simulink model "test_nlin_interp2"  (R2015a)
settings: Solver=ode45  StartTime=0.0  StopTime=u(end,1)  FixedStep=0.001  RelTol=1e-6
PostLoadFcn:
  | , if any(exist('dsrtsu_mdlpostloadfcn', 'file') == [2, 3, 6]), try dsrtsu_mdlpostloadfcn('Execute', bdroot); catch fprintf('Error in PostLoadFcn (dsrtsu_mdlpostloadfcn) for model "%s":\n %s\n', bdroot, lasterr); end, end,
values from neighbouring files (symbols this model uses):
  c = rectangle('Parent',ax)    [DoublePendulum.m]    (also in init.m = 2.99880047981; interpolate.m = 2.99880047981; plot_17.m = 2.99880047981)
  g = 9.81    [init.m]    (also in interpolate.m; plot_17.m; plot_generic.m)
  T1 = 0.0395    [init.m]    (also in interpolate.m = 0.025; plot_17.m = 0.025; plot_generic.m)
settings Model: DSRTSU_INTERNAL_RTI_VER=360  DSRTSU_INTERNAL_RTI_TYPE=rti1104  CovSFcnEnable=off  Creator=labor  LastModifiedBy=Schuettler
settings DataIOCC: LimitDataPoints=off  SignalLoggingSaveFormat=ModelDataLogs
settings OptimizationCC: BlockReduction=off  OptimizeBlockIOStorage=off  BufferReuse=off  GlobalBufferReuse=off  ExpressionFolding=off  ExpressionDepthLimit=2147483647  LocalBlockOutputs=off  InitFltsAndDblsToZero=on  OptimizeModelRefInitCode=on  LifeSpan=1
settings DebuggingCC: UnderspecifiedInitializationDetection=Classic  MergeDetectMultiDrivingBlocksExec=none  SolverPrmCheckMsg=warning  FcnCallInpInsideContextMsg=UseLocalSettings  StateNameClashWarn=warning
settings HardwareCC: ProdIntDivRoundTo=Zero  ProdEndianess=BigEndian  ProdHWDeviceType=Generic->Custom  TargetIntDivRoundTo=Zero  TargetEndianess=BigEndian  TargetHWDeviceType=Generic->Custom
settings RTWCC: SystemTargetFile=ert.tlc  TemplateMakefile=ert_default_tmf  Description=Embedded Coder
settings CodeAppCC: IgnoreCustomStorageClasses=off
settings ERTTargetCC: ParMdlRefBuildCompliant=on  CompOptLevelCompliant=on  ConcurrentExecutionCompliant=on  ERTFirstTimeCompliant=on  SupportContinuousTime=off  SupportVariableSizeSignals=off  ModelStepFunctionPrototypeControlCompliant=on  CPPClassGenCompliant=on  InlinedParameterPlacement=Hierarchical  ERTCustomFileTemplate=example_file_process.tlc

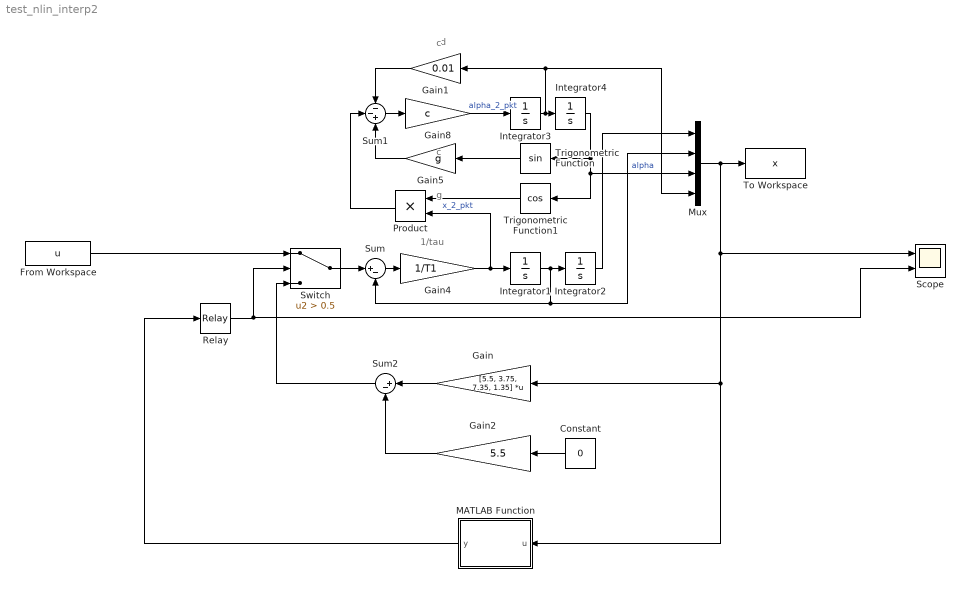
== system test_nlin_interp2 ==
  note: d
  note: 1/tau
  note: g
  note: c
  note: c
  Constant : Constant  Value=0
  From Workspace : FromWorkspace  VariableName=u  SampleTime=0
  Gain : Gain  Gain=[5.5, 3.75, 7.35, 1.35]  Multiplication=Matrix(K*u) (u vector)
  Gain1 : Gain  Gain=0.01
  Gain2 : Gain  Gain=5.5
  Gain4 : Gain  Gain=1/T1
  Gain5 : Gain  Gain=g
  Gain8 : Gain  Gain=c
  Integrator1 : Integrator
  Integrator2 : Integrator
  Integrator3 : Integrator
  Integrator4 : Integrator  InitialCondition=pi
  MATLAB Function : MATLAB Function  TreatAsAtomicUnit=on
  Mux : Mux
  Product : Product  RndMeth=Zero
  Relay : Relay  OnSwitchValue=0.17  OffSwitchValue=0.02
  Scope : Scope  NumInputPorts=2
      settings: YMin=-5~-5  YMax=5~5
  Sum : Sum  Inputs=|+-
  Sum1 : Sum  Inputs=--+
  Sum2 : Sum  Inputs=|+-
  Switch : Switch  Criteria=u2 > Threshold  Threshold=0.5
  To Workspace : ToWorkspace  VariableName=x  SampleTime=-1
  Trigonometric Function : Trigonometry
  Trigonometric Function1 : Trigonometry  Operator=cos
  wires:
  Integrator1/1 -> Sum/2, Mux/2, Integrator2/1
  Integrator3/1 -> Mux/4, Gain1/1, Integrator4/1
  Gain4/1 -> Integrator1/1, Product/2  "x_2_pkt"
  Sum/1 -> Gain4/1
  Trigonometric Function1/1 -> Product/1
  Sum1/1 -> Gain8/1
  Gain8/1 -> Integrator3/1  "alpha_2_pkt"
  Integrator4/1 -> Mux/3, Trigonometric Function1/1, Trigonometric Function/1  "alpha"
  Integrator2/1 -> Mux/1
  Trigonometric Function/1 -> Gain5/1
  Gain5/1 -> Sum1/3
  Product/1 -> Sum1/2
  Gain1/1 -> Sum1/1
  Mux/1 -> Scope/1, MATLAB Function/1(u), Gain/1, To Workspace/1
  From Workspace/1 -> Switch/1
  Gain/1 -> Sum2/1
  Gain2/1 -> Sum2/2
  Constant/1 -> Gain2/1
  Switch/1 -> Sum/1
  Sum2/1 -> Switch/3
  MATLAB Function/1(y) -> Relay/1
  Relay/1 -> Switch/2, Scope/2

== matlab function test_nlin_interp2/MATLAB Function ==
  data: u input; y output
function y = fcn(u)

weight1 = [1.37405, 0.0, 0.040207, 0.0];
weight2 = 0.002639;
l = 0.5;
gl = 9.81*l;
J_eff = (4.0*l*l + 0.02*0.02) / 12.0;
    
x = u;
x(3) = mod(x(3)+pi,2*pi)-pi;
E = (cos(x(3)) - 1)*(x(2)*x(4)*l+gl)+x(4)^2*J_eff+x(2)^2;

y = (x.^2)'*weight1' + E^2*weight2;
